simulink model "Exe1_CAM"  (R2024b)
settings: Solver=VariableStepAuto  StartTime=0.0  StopTime=T_sim  RelTol=1e-3
values from neighbouring files (symbols this model uses):
  C1 = 5    [Exe1_CAM_main.m]
  C2 = 1    [Exe1_CAM_main.m]
  h1_ini = 0.7    [Exe1_CAM_main.m]
  h1_ref = 1    [Exe1_CAM_main.m]
  h2_ini = 0.6    [Exe1_CAM_main.m]
  h2_ref = 1.2    [Exe1_CAM_main.m]
  u1_max = 0.9    [Exe1_CAM_main.m]
  u1_min = 0    [Exe1_CAM_main.m]
  u1_ref = k*sqrt(h2_ref)    [Exe1_CAM_main.m]
  u2_max = 0.9    [Exe1_CAM_main.m]
  u2_min = 0    [Exe1_CAM_main.m]
  u2_ref = u1_ref    [Exe1_CAM_main.m]
libraries: cstblocks x1
settings Model: Creator=luca.zucchetti  LastModifiedBy=luca.zucchetti

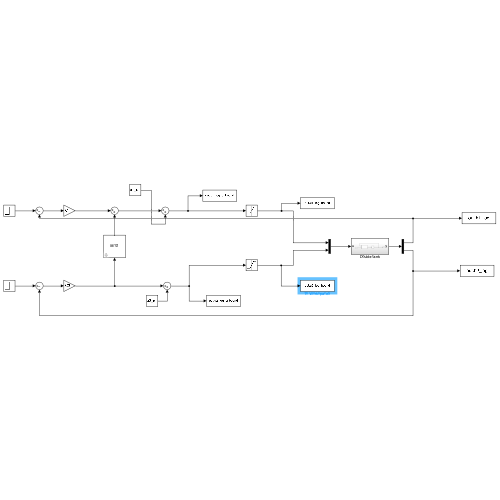
[thumbnail: Simulink's stored preview of the top-level diagram]
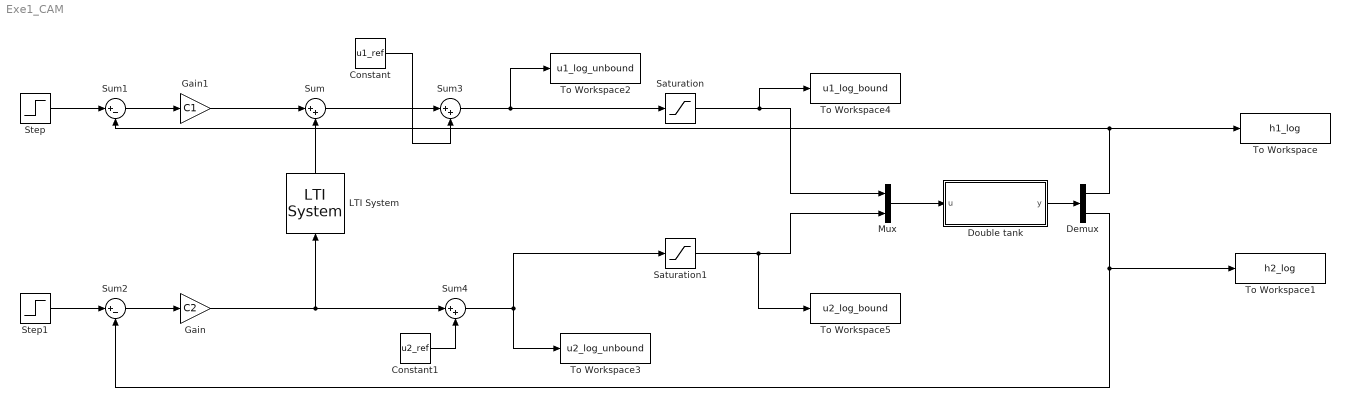
== system Exe1_CAM ==
  Constant : Constant  Value=u1_ref
  Constant1 : Constant  Value=u2_ref
  Demux : Demux  Outputs=2
  Double tank : Subsystem
  Gain : Gain  Gain=C2
  Gain1 : Gain  Gain=C1
  LTI System : cstblocks/LTI System  sys=M12  IC=[]  PadeOrder=0
  Mux : Mux  Inputs=2
  Saturation : Saturate  UpperLimit=u1_max  LowerLimit=u1_min
  Saturation1 : Saturate  UpperLimit=u2_max  LowerLimit=u2_min
  Step : Step  Before=h1_ini  After=h1_ref  SampleTime=0
  Step1 : Step  Before=h2_ini  After=h2_ref  SampleTime=0
  Sum : Sum  Inputs=|++
  Sum1 : Sum  Inputs=|+-
  Sum2 : Sum  Inputs=|+-
  Sum3 : Sum  Inputs=|++
  Sum4 : Sum  Inputs=|++
  To Workspace : ToWorkspace  VariableName=h1_log  SaveFormat=Timeseries  SampleTime=-1
  To Workspace1 : ToWorkspace  VariableName=h2_log  SaveFormat=Timeseries  SampleTime=-1
  To Workspace2 : ToWorkspace  VariableName=u1_log_unbound  SaveFormat=Timeseries  SampleTime=-1
  To Workspace3 : ToWorkspace  VariableName=u2_log_unbound  SaveFormat=Timeseries  SampleTime=-1
  To Workspace4 : ToWorkspace  VariableName=u1_log_bound  SaveFormat=Timeseries  SampleTime=-1
  To Workspace5 : ToWorkspace  VariableName=u2_log_bound  SaveFormat=Timeseries  SampleTime=-1
  wires:
  Gain1/1 -> Sum/1
  LTI System/1 -> Sum/2
  Double tank/1(y) -> Demux/1
  Step/1 -> Sum1/1
  Step1/1 -> Sum2/1
  Sum1/1 -> Gain1/1
  Sum2/1 -> Gain/1
  Demux/1 -> To Workspace/1, Sum1/2
  Demux/2 -> To Workspace1/1, Sum2/2
  Gain/1 -> Sum4/1, LTI System/1
  Sum/1 -> Sum3/1
  Constant/1 -> Sum3/2
  Sum3/1 -> Saturation/1, To Workspace2/1
  Constant1/1 -> Sum4/2
  Sum4/1 -> Saturation1/1, To Workspace3/1
  Mux/1 -> Double tank/1(u)
  Saturation/1 -> To Workspace4/1, Mux/1
  Saturation1/1 -> To Workspace5/1, Mux/2

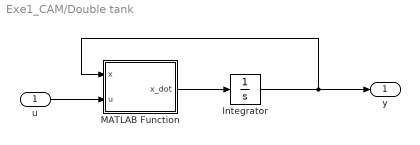
== system Exe1_CAM/Double tank ==
  u : Inport
  Integrator : Integrator  InitialCondition=[h1_ini; h2_ini]
  MATLAB Function : MATLAB Function  TreatAsAtomicUnit=on
  y : Outport
  wires:
  u/1 -> MATLAB Function/2(u)
  MATLAB Function/1(x_dot) -> Integrator/1
  Integrator/1 -> MATLAB Function/1(x), y/1

== matlab function Exe1_CAM/Double tank/MATLAB Function ==
  data: x input; u input; x_dot output; k parameter
function x_dot = double_tank(x, u, k)
x_dot = zeros(2,1); %inizializzo a zeri un vettore colonna di due righe

x_dot(1) = u(1) - u(2);
x_dot(2) = u(2) - k*sqrt(x(2));
